simulink model "scon2_L9_1ponto2_simulink"  (R2024a)
settings: Solver=VariableStepAuto  StartTime=0.0  StopTime=10.0  RelTol=1e-3
values from neighbouring files (symbols this model uses):
  A = [0, 1, 0; 0, 0, 1; -8, -3, -3]    [scon2_L9_1ponto2.m]
  B = [0; 0; 4]    [scon2_L9_1ponto2.m]
  C = [2, -9, 2]    [scon2_L9_1ponto2.m]
  K = acker(A, B, J_c)    [scon2_L9_1ponto2.m]
  K_e = acker(A', C', J_o)'    [scon2_L9_1ponto2.m]
  x0 = [1; 2; 3]    [scon2_L9_1ponto2.m]
settings Model: Creator=Carlos Augusto  LastModifiedBy=Carlos Augusto

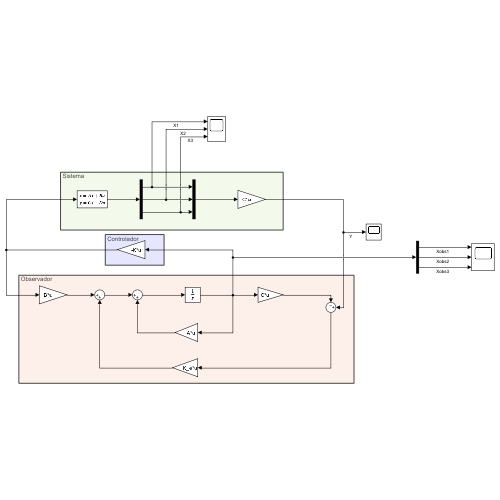
[thumbnail: Simulink's stored preview of the top-level diagram]
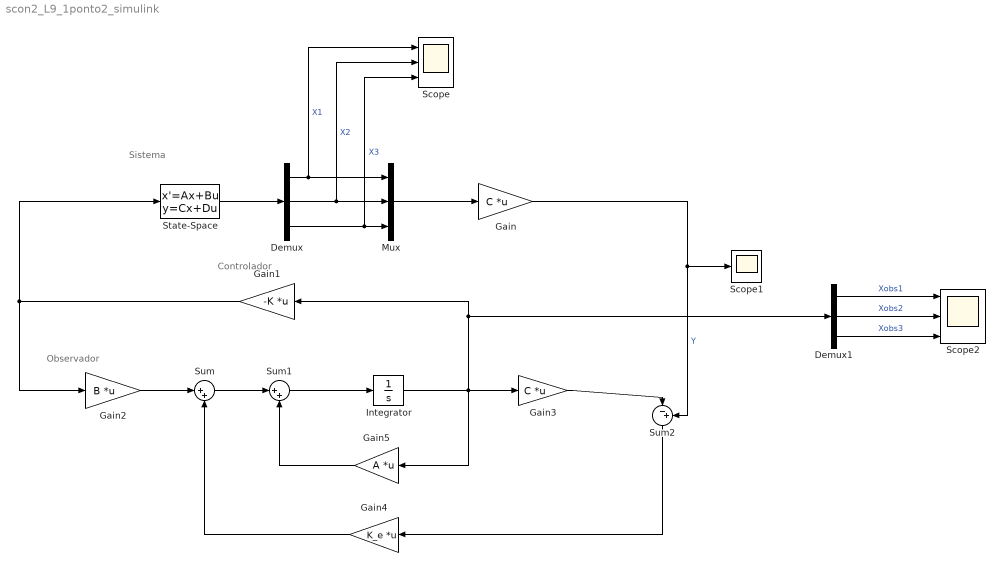
== system scon2_L9_1ponto2_simulink ==
  note: Observador
  note: Controlador
  note: Sistema
  Demux : Demux  Outputs=3
  Demux1 : Demux  Outputs=3
  Gain : Gain  Gain=C  Multiplication=Matrix(K*u)
  Gain1 : Gain  Gain=-K  Multiplication=Matrix(K*u)
  Gain2 : Gain  Gain=B  Multiplication=Matrix(K*u)
  Gain3 : Gain  Gain=C  Multiplication=Matrix(K*u)
  Gain4 : Gain  Gain=K_e  Multiplication=Matrix(K*u)
  Gain5 : Gain  Gain=A  Multiplication=Matrix(K*u)
  Integrator : Integrator
  Mux : Mux  Inputs=3
  Scope : Scope  NumInputPorts=3
  Scope1 : Scope
  Scope2 : Scope  NumInputPorts=3
  State-Space : StateSpace  A=A  B=B  C=eye(3)  D=zeros(3, 1)  InitialCondition=x0
  Sum : Sum  Inputs=|++
  Sum1 : Sum  Inputs=|++
  Sum2 : Sum  Inputs=|-+
  wires:
  State-Space/1 -> Demux/1
  Demux/1 -> Mux/1, Scope/1  "X1"
  Demux/2 -> Mux/2, Scope/2  "X2"
  Demux/3 -> Mux/3, Scope/3  "X3"
  Mux/1 -> Gain/1
  Gain1/1 -> Gain2/1, State-Space/1
  Gain2/1 -> Sum/1
  Sum/1 -> Sum1/1
  Sum1/1 -> Integrator/1
  Integrator/1 -> Gain1/1, Demux1/1, Gain5/1, Gain3/1
  Gain3/1 -> Sum2/1
  Gain4/1 -> Sum/2
  Sum2/1 -> Gain4/1
  Gain/1 -> Scope1/1, Sum2/2  "Y"
  Gain5/1 -> Sum1/2
  Demux1/1 -> Scope2/1  "Xobs1"
  Demux1/2 -> Scope2/2  "Xobs2"
  Demux1/3 -> Scope2/3  "Xobs3"
